simulink model "DTC"  (R2018b)
settings: Solver=ode23tb  StartTime=0.0  StopTime=0.4  RelTol=1e-4
InitFcn:
  | A = [5 6 1 2 3 4;3 4 5 6 1 2;6 1 2 3 4 5;2 3 4 5 6 1];
  | states = [1 0 0;1 1 0;0 1 0;0 1 1;0 0 1;1 0 1];
libraries: powerlib x6
settings Model: Creator=123  LastModifiedBy=123

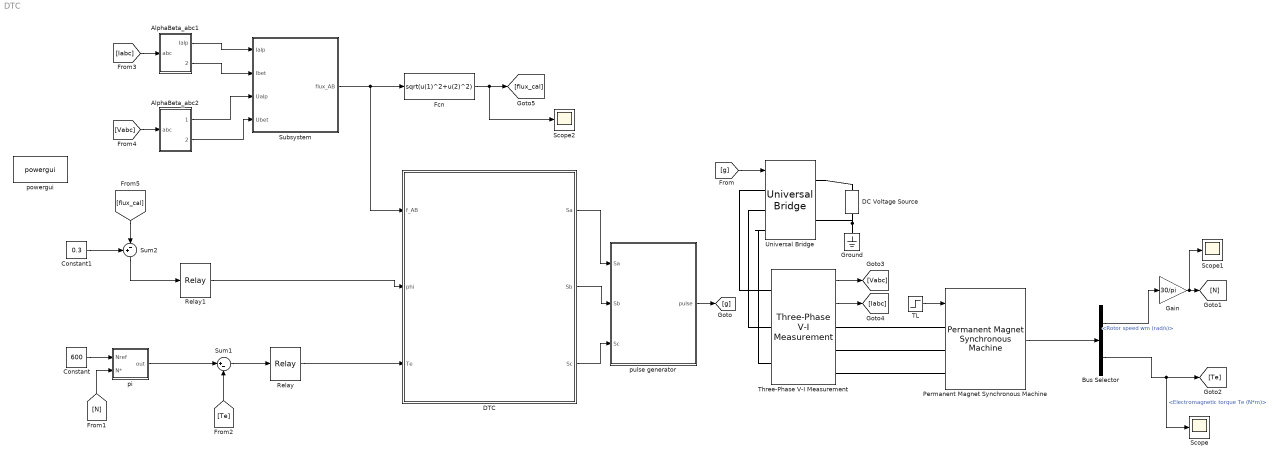
== system DTC ==
  AlphaBeta_abc1 : Subsystem
  AlphaBeta_abc2 : Subsystem
  Bus Selector : BusSelector  OutputSignals=Rotor speed wm (rad/s),Electromagnetic torque Te (N*m)
  Constant : Constant  Value=600
  Constant1 : Constant  Value=0.3
  DC Voltage Source : powerlib/Electrical Sources/DC Voltage Source  Amplitude=311  Measurements=None
      settings: SourceProductName=Simscape Electrical
  DTC : MATLAB Function  TreatAsAtomicUnit=on
  Fcn : Fcn  Expr=sqrt(u(1)^2+u(2)^2)
  Gain : Gain  Gain=30/pi
  Ground : powerlib/Elements/Ground  LConnTagsString=a
  Permanent Magnet Synchronous Machine : powerlib/Machines/Permanent Magnet Synchronous Machine  NbPhases=3  FluxDistribution=Sinusoidal  RotorType=Round  MechanicalLoad=Torque Tm  PresetModel=No  ShowDetailedParameters=on  MeasurementBus=off  Resistance=1.2  Inductance=8.5e-3  dqInductances=[4e-3,6e-3]  La=8.5e-3  MachineConstant=Flux linkage established by magnets (V.s)  Flux=0.175  VoltageCst=126.966  TorqueCst=1.05  Flat=120  Mechanical=[0.0008 0 4 0]  PolePairs=4  InitialConditions=[0,0, 0,0]  InitialConditions5ph=[0 0 0 0 0 0]  TsPowergui=0  TsBlock=-1  RefAngle=Aligned with phase A axis (original Park)
  Relay : Relay  OnSwitchValue=0.1  OffSwitchValue=-0.1
  Relay1 : Relay  OnSwitchValue=0.002  OffSwitchValue=-0.002
  Scope : Scope
  Scope1 : Scope
  Scope2 : Scope
  Subsystem : Subsystem
  Sum1 : Sum  Inputs=|+-
  Sum2 : Sum  Inputs=+-|
  TL : Step  Time=0.2  After=2  SampleTime=2.5e-6
  Three-Phase V-I Measurement : powerlib/Measurements/Three-Phase V-I Measurement  VoltageMeasurement=phase-to-ground  SetLabelV=off  LabelV=Vabc  Vpu=off  VpuLL=off  CurrentMeasurement=yes  SetLabelI=off  LabelI=Iabc  Ipu=off  Pbase=100e6  Vbase=500e3  OutputType=Complex  PhasorSimulation=off  PSBequivalent=0
  Universal Bridge : powerlib/Power Electronics/Universal Bridge  Arms=3  SnubberResistance=1e5  SnubberCapacitance=inf  Device=IGBT / Diodes  Ron=1e-3  Lon=0  ForwardVoltages="[  0  0  ]"  ForwardVoltage=0  GTOparameters=[ 10e-6 , 20e-6 ]  IGBTparameters=[ 1e-6 , 2e-6 ]  Measurements=None  Measurements_2=None  converterType=Rectifier
      settings: SourceProductName=Simscape Electrical
  pi : Subsystem
  powergui : powerlib/powergui  Priority=1  SimulationMode=Discrete  SampleTime=5e-6  frequency=60  Iterations=50  frequencyindice=0  Pbase=100e6  ErrMax=1e-4  UnitsV=kV  UnitsW=MW  buscounter=0  FunctionMessages=off  echomessages=off  EnableUseOfTLC=off  CurrentSourceSwitches=off  DisableSnubberDevices=off  DisableRonSwitches=off  DisableVfSwitches=off  DisplayEquations=off  SolverType=Tustin/Backward Euler (TBE)  Interpol=off  ExternalGateDelay=off  methode=off  Ts=100  x0status=blocks  SPID=on  SwTol=0  HookPort=off  RestoreLinks=warning  ResistiveCurrentMeasurement=off  Frange=[0:2:500]  Ylog=off  Xlog=on  ShowGrid=off  save=off  variable=ZData  structure=0  ZoomFFT=off  StartTime=0.0  cycles=1  DisplayStyle=1  fundamental=60  FreqAxis=off  MaxFrequency=1000  frequencyindicesteady=1  RmsSteady=1  display=off
  pulse generator : Subsystem
  wires:
  [g] -> Universal Bridge/1
  Bus Selector/1 -> Gain/1  "<Rotor speed wm (rad/s)>"
  Constant/1 -> pi/1(Nref)
  [N] -> pi/2(N*)
  Gain/1 -> Scope1/1, [N]
  [Te] -> Sum1/2
  Bus Selector/2 -> Scope/1, [Te]  "<Electromagnetic torque Te (N*m)>"
  Sum1/1 -> Relay/1
  Sum2/1 -> Relay1/1
  Constant1/1 -> Sum2/1
  Three-Phase V-I Measurement/2 -> [Iabc]
  Three-Phase V-I Measurement/1 -> [Vabc]
  Relay/1 -> DTC/3(Te)
  Relay1/1 -> DTC/2(phi)
  [Iabc] -> AlphaBeta_abc1/1(abc)
  [Vabc] -> AlphaBeta_abc2/1(abc)
  AlphaBeta_abc1/1(Ialp) -> Subsystem/1(Ialp)
  AlphaBeta_abc1/2(Ibet) -> Subsystem/2(Ibet)
  AlphaBeta_abc2/1(Ualp) -> Subsystem/3(Ualp)
  AlphaBeta_abc2/2(Ubet) -> Subsystem/4(Ubet)
  Subsystem/1(flux_AB) -> Fcn/1, DTC/1(f_AB)
  Fcn/1 -> Scope2/1, [flux_cal]
  [flux_cal] -> Sum2/2
  DTC/1(Sa) -> pulse generator/1(Sa)
  DTC/2(Sb) -> pulse generator/2(Sb)
  DTC/3(Sc) -> pulse generator/3(Sc)
  pulse generator/1(pulse) -> [g]
  pi/1(out) -> Sum1/1
  Permanent Magnet Synchronous Machine/1 -> Bus Selector/1
  TL/1 -> Permanent Magnet Synchronous Machine/1
  connections:
  Universal Bridge/RConn1 -- DC Voltage Source/RConn1
  DC Voltage Source/LConn1 -- Universal Bridge/RConn2 -- Ground/LConn1
  Universal Bridge/LConn1 -- Three-Phase V-I Measurement/LConn1
  Universal Bridge/LConn2 -- Three-Phase V-I Measurement/LConn2
  Universal Bridge/LConn3 -- Three-Phase V-I Measurement/LConn3
  Three-Phase V-I Measurement/RConn1 -- Permanent Magnet Synchronous Machine/LConn1
  Three-Phase V-I Measurement/RConn2 -- Permanent Magnet Synchronous Machine/LConn2
  Three-Phase V-I Measurement/RConn3 -- Permanent Magnet Synchronous Machine/LConn3

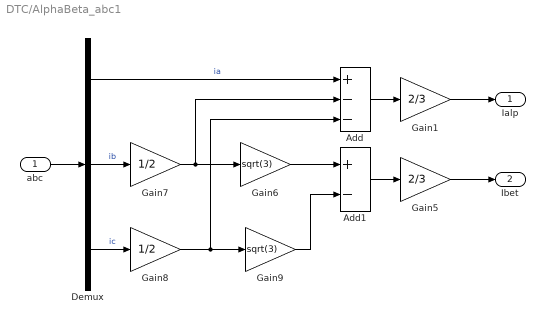
== system DTC/AlphaBeta_abc1 ==
  abc : Inport
  Add : Sum  Inputs=+--
  Add1 : Sum  Inputs=+-
  Demux : Demux  Outputs=3
  Gain1 : Gain  Gain=2/3
  Gain5 : Gain  Gain=2/3
  Gain6 : Gain  Gain=sqrt(3)
  Gain7 : Gain  Gain=1/2
  Gain8 : Gain  Gain=1/2
  Gain9 : Gain  Gain=sqrt(3)
  Ialp : Outport
  Ibet : Outport  Port=2
  wires:
  abc/1 -> Demux/1
  Demux/2 -> Gain7/1  "ib"
  Demux/3 -> Gain8/1  "ic"
  Add/1 -> Gain1/1
  Gain7/1 -> Gain6/1, Add/2
  Gain8/1 -> Gain9/1, Add/3
  Gain6/1 -> Add1/1
  Gain9/1 -> Add1/2
  Demux/1 -> Add/1  "ia"
  Add1/1 -> Gain5/1
  Gain1/1 -> Ialp/1
  Gain5/1 -> Ibet/1

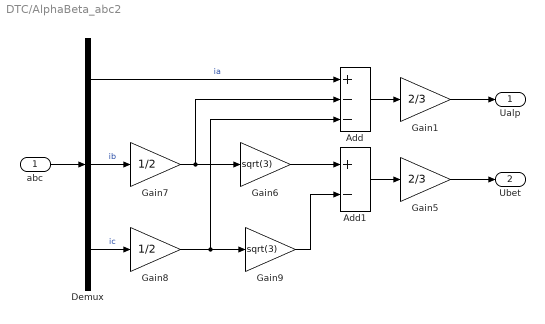
== system DTC/AlphaBeta_abc2 ==
  abc : Inport
  Add : Sum  Inputs=+--
  Add1 : Sum  Inputs=+-
  Demux : Demux  Outputs=3
  Gain1 : Gain  Gain=2/3
  Gain5 : Gain  Gain=2/3
  Gain6 : Gain  Gain=sqrt(3)
  Gain7 : Gain  Gain=1/2
  Gain8 : Gain  Gain=1/2
  Gain9 : Gain  Gain=sqrt(3)
  Ualp : Outport
  Ubet : Outport  Port=2
  wires:
  Gain5/1 -> Ubet/1
  Gain1/1 -> Ualp/1
  Add1/1 -> Gain5/1
  Demux/1 -> Add/1  "ia"
  Gain9/1 -> Add1/2
  Gain6/1 -> Add1/1
  Gain8/1 -> Add/3, Gain9/1
  Gain7/1 -> Add/2, Gain6/1
  Add/1 -> Gain1/1
  Demux/3 -> Gain8/1  "ic"
  Demux/2 -> Gain7/1  "ib"
  abc/1 -> Demux/1

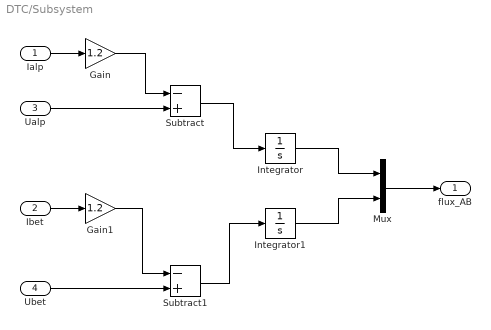
== system DTC/Subsystem ==
  Ialp : Inport
  Ibet : Inport  Port=2
  Ualp : Inport  Port=3
  Ubet : Inport  Port=4
  Gain : Gain  Gain=1.2
  Gain1 : Gain  Gain=1.2
  Integrator : Integrator  InitialCondition=0.11
  Integrator1 : Integrator  InitialCondition=0.11
  Mux : Mux  Inputs=2
  Subtract : Sum  Inputs=-+
  Subtract1 : Sum  Inputs=-+
  flux_AB : Outport
  wires:
  Ialp/1 -> Gain/1
  Gain/1 -> Subtract/1
  Ualp/1 -> Subtract/2
  Ibet/1 -> Gain1/1
  Ubet/1 -> Subtract1/2
  Gain1/1 -> Subtract1/1
  Subtract/1 -> Integrator/1
  Subtract1/1 -> Integrator1/1
  Integrator/1 -> Mux/1
  Integrator1/1 -> Mux/2
  Mux/1 -> flux_AB/1

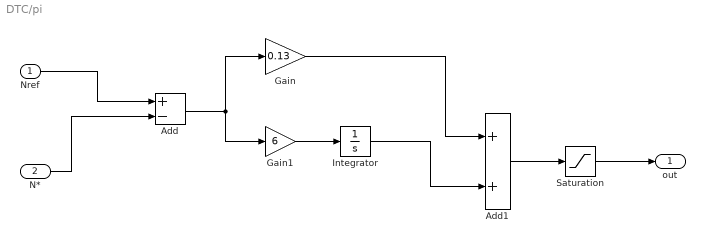
== system DTC/pi ==
  Nref : Inport
  N* : Inport  Port=2
  Add : Sum  Inputs=+-
  Add1 : Sum
  Gain : Gain  Gain=0.13
  Gain1 : Gain  Gain=6
  Integrator : Integrator
  Saturation : Saturate  UpperLimit=20  LowerLimit=-20
  out : Outport
  wires:
  Nref/1 -> Add/1
  N*/1 -> Add/2
  Add/1 -> Gain1/1, Gain/1
  Gain/1 -> Add1/1
  Gain1/1 -> Integrator/1
  Integrator/1 -> Add1/2
  Add1/1 -> Saturation/1
  Saturation/1 -> out/1

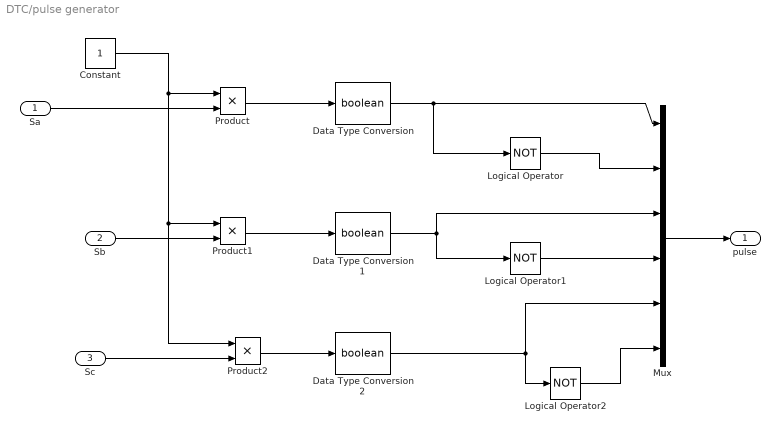
== system DTC/pulse generator ==
  Sa : Inport
  Sb : Inport  Port=2
  Sc : Inport  Port=3
  Constant : Constant  SampleTime=-1
  Data Type Conversion : DataTypeConversion  OutDataTypeStr=boolean
  Data Type Conversion1 : DataTypeConversion  OutDataTypeStr=boolean
  Data Type Conversion2 : DataTypeConversion  OutDataTypeStr=boolean
  Logical Operator : Logic  Operator=NOT  AllPortsSameDT=off
  Logical Operator1 : Logic  Operator=NOT  AllPortsSameDT=off
  Logical Operator2 : Logic  Operator=NOT  AllPortsSameDT=off
  Mux : Mux  Inputs=6
  Product : Product
  Product1 : Product
  Product2 : Product
  pulse : Outport
  wires:
  Sa/1 -> Product/2
  Sb/1 -> Product1/2
  Constant/1 -> Product2/1, Product1/1, Product/1
  Product/1 -> Data Type Conversion/1
  Product1/1 -> Data Type Conversion1/1
  Logical Operator/1 -> Mux/2
  Data Type Conversion/1 -> Mux/1, Logical Operator/1
  Logical Operator1/1 -> Mux/4
  Data Type Conversion1/1 -> Mux/3, Logical Operator1/1
  Mux/1 -> pulse/1
  Sc/1 -> Product2/2
  Product2/1 -> Data Type Conversion2/1
  Logical Operator2/1 -> Mux/6
  Data Type Conversion2/1 -> Mux/5, Logical Operator2/1

== matlab function DTC/DTC ==
  data: f_AB input; Sa output; phi input; Te input; A parameter; states parameter; Sb output; Sc output
function [Sa,Sb,Sc]  = control(f_AB,phi,Te,A,states)
F = f_AB(1) + 1j*f_AB(2);
th = angle(F);
th1=mod(th+pi/6,2*pi);
N = floor(th1/(pi/3)) + 1;
if N>6
    N = 1;
end

c = phi*2 + Te + 1;
% c = min(max(c,1),4);
m = A(c,N);
% m = min(max(m,1),6);
Sa = states(m,1);
Sb = states(m,2);
Sc = states(m,3);
